simulink model "test9_sub_named_Simulink_orig"  (R2016b)
settings: Solver=VariableStepAuto  StartTime=0.0  StopTime=10.0  RelTol=1e-3
settings Model: Creator=gm  LastModifiedBy=gm

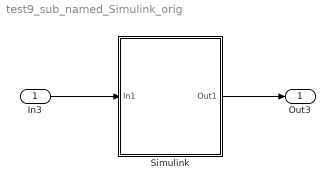
== system test9_sub_named_Simulink_orig ==
  In3 : Inport
  Simulink : Subsystem
  Out3 : Outport
  wires:
  In3/1 -> Simulink/1(In1)
  Simulink/1(Out1) -> Out3/1

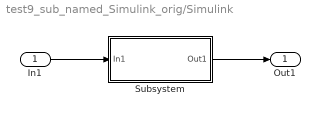
== system test9_sub_named_Simulink_orig/Simulink ==
  In1 : Inport
  Subsystem : Subsystem
  Out1 : Outport
  wires:
  In1/1 -> Subsystem/1(In1)
  Subsystem/1(Out1) -> Out1/1

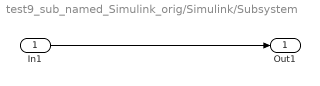
== system test9_sub_named_Simulink_orig/Simulink/Subsystem ==
  In1 : Inport
  Out1 : Outport
  wires:
  In1/1 -> Out1/1
